simulink model "sldemo_varsize_multimode"  (Simulink 7.6)
settings: Solver=FixedStepDiscrete  StartTime=0.0  StopTime=20  RelTol=1e-3
libraries: simulink x4
settings Model: Creator=The MathWorks Inc.
settings OptimizationCC: InitFltsAndDblsToZero=on
settings SFSimCC: SimParseCustomCode=off

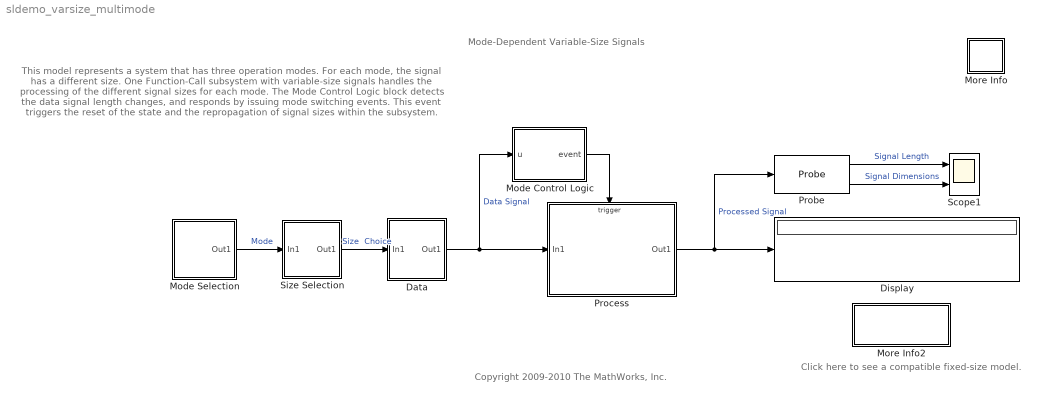
== system sldemo_varsize_multimode ==
  note: Mode-Dependent Variable-Size Signals
  note: Copyright 2009-2010 The MathWorks, Inc.
  note: This model represents a system that has three operation modes. For each mode, the signal has a different size.
      | One Function-Call subsystem with variable-size signals handles the processing of the different signal sizes for each mode. The
      | Mode Control Logic block detects the data signal length changes, and responds by issuing mode switching events. This event
      | triggers the reset of the state and the repropagation of signal sizes within the subsystem.
  note: Click here to see a compatible
      | fixed-size model.
  Data : Subsystem
  Display : Display
  Mode Control Logic : Stateflow chart  TreatAsAtomicUnit=on
  "Mode Selection " : Subsystem
  More Info : Subsystem
      settings: OpenFcn=showdemo(bdroot(gcb))
      mask Display: disp('?')
  More Info2 : Subsystem
      settings: OpenFcn=sldemo_varsize_multimodeFixSizeImpl
      mask Display: disp('Fixed-Size Signal\nImplementation')
  Probe : Probe  ProbeSampleTime=off  ProbeComplexSignal=off  ProbeSignalDimensions=on
  Process : Subsystem  TreatAsAtomicUnit=on
  Scope1 : Scope  NumInputPorts=2
      settings: TimeRange=20  YMin=0~0.5  YMax=10~3.5
  Size Selection : Subsystem
  wires:
  Data/1(Out1) -> Mode Control Logic/1(u), Process/1(In1)  "Data Signal"
  "Mode Selection "/1(Out1) -> Size Selection/1(In1)  "Mode"
  Size Selection/1(Out1) -> Data/1(In1)  "Size  Choice"
  Probe/1 -> Scope1/1  "Signal Length"
  Mode Control Logic/1(event) -> Process/Trigger
  Probe/2 -> Scope1/2  "Signal Dimensions"
  Process/1(Out1) -> Display/1, Probe/1  "Processed Signal"

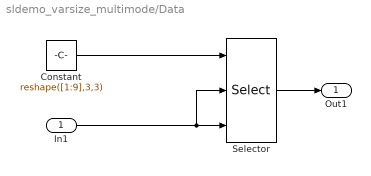
== system sldemo_varsize_multimode/Data ==
  In1 : Inport
  Constant : Constant  Value=reshape([1:9],3,3)
  Selector : Selector  NumberOfDimensions=2  InputPortWidth=3  IndexOptions=Starting and ending indices (port),Starting and ending indices (port)  Indices=[1 3],1  OutputSizes=1,1
  Out1 : Outport
  wires:
  Constant/1 -> Selector/1
  Selector/1 -> Out1/1
  In1/1 -> Selector/3, Selector/2

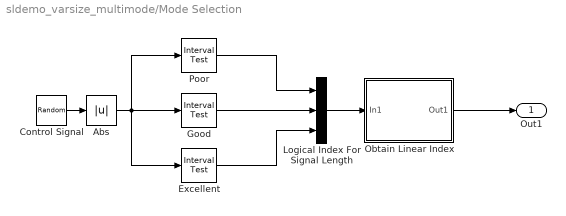
== system sldemo_varsize_multimode/Mode Selection  ==
  Abs : Abs
  Control Signal : RandomNumber  Variance=0.25  SampleTime=1
  Excellent : simulink/Logic and Bit Operations/Interval Test  SystemSampleTime=-1  IntervalClosedRight=off  uplimit=inf  IntervalClosedLeft=on  lowlimit=0.50  LogicOutDataTypeMode=uint8
  Good : simulink/Logic and Bit Operations/Interval Test  SystemSampleTime=-1  IntervalClosedRight=off  uplimit=0.50  IntervalClosedLeft=on  lowlimit=0.25  LogicOutDataTypeMode=uint8
  Logical Index For Signal Length : Concatenate  NumInputs=3  Mode=Vector
  Obtain Linear Index : Subsystem
  Poor : simulink/Logic and Bit Operations/Interval Test  SystemSampleTime=-1  IntervalClosedRight=off  uplimit=0.25  IntervalClosedLeft=on  lowlimit=0.0  LogicOutDataTypeMode=uint8
  Out1 : Outport
  wires:
  Logical Index For Signal Length/1 -> Obtain Linear Index/1(In1)
  Poor/1 -> Logical Index For Signal Length/1
  Excellent/1 -> Logical Index For Signal Length/3
  Good/1 -> Logical Index For Signal Length/2
  Abs/1 -> Excellent/1, Poor/1, Good/1
  Obtain Linear Index/1(Out1) -> Out1/1
  Control Signal/1 -> Abs/1

== system sldemo_varsize_multimode/More Info ==
  note: Bus Block Demonstration
  note: This demonstration shows how signals may be grouped and ungrouped while
      | retaining their names.  In this demonstration, 5 signals are created and labelled
      | appropriately.  These signals are then mux'd together to create a bus of signals.
      | This bus of signals is then fed into the Bus Selector block.  Inside of the Bus
      | Selector block, the Pulse and Chirp signals are chosen to be output from the
      | original signal bus.
      |
      | It is possible to place a nest signal buses and then still retrieve the original signal
      | with its label.

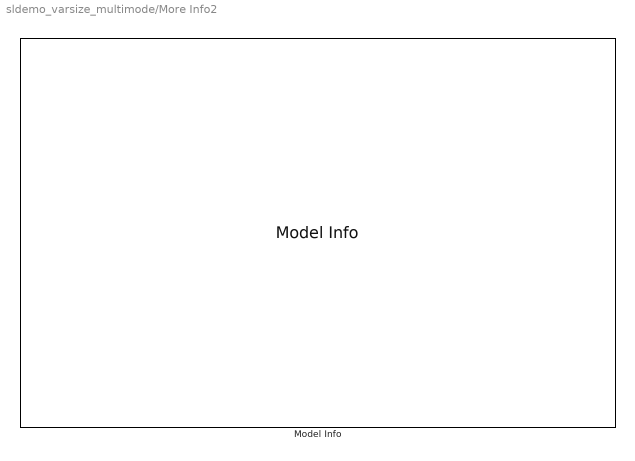
== system sldemo_varsize_multimode/More Info2 ==
  Model Info : simulink/Model-Wide Utilities/Model Info  SystemSampleTime=-1  InitialBlockCM=None  BlockCM=none  Frame=on  DisplayStringWithTags=Model Info  HorizontalTextAlignment=Left  LeftAlignmentValue=0.02  SourceBlockDiagram=sldemo_varsize_multimode  TagMaxNumber=20

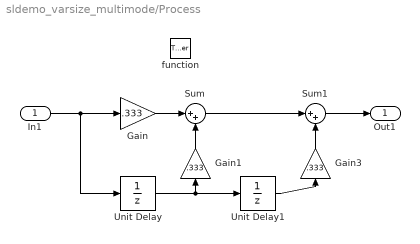
== system sldemo_varsize_multimode/Process ==
  In1 : Inport
  function : TriggerPort  TriggerType=function-call  StatesWhenEnabling=reset  PropagateVarSize=Only when enabling  SampleTimeType=periodic
  Gain : Gain  Gain=.333
  Gain1 : Gain  Gain=.333
  Gain3 : Gain  Gain=.333
  Sum : Sum  Inputs=|++
  Sum1 : Sum  Inputs=|++
  Unit Delay : UnitDelay  SampleTime=-1
  Unit Delay1 : UnitDelay  SampleTime=-1
  Out1 : Outport
  wires:
  Unit Delay/1 -> Gain1/1, Unit Delay1/1
  Gain/1 -> Sum/1
  Gain1/1 -> Sum/2
  In1/1 -> Gain/1, Unit Delay/1
  Unit Delay1/1 -> Gain3/1
  Gain3/1 -> Sum1/2
  Sum/1 -> Sum1/1
  Sum1/1 -> Out1/1

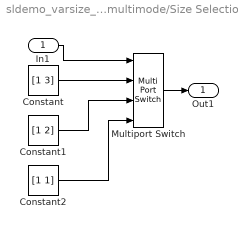
== system sldemo_varsize_multimode/Size Selection ==
  In1 : Inport
  Constant : Constant  Value=[1 3]
  Constant1 : Constant  Value=[1 2]
  Constant2 : Constant  Value=[1 1]
  Multiport Switch : MultiPortSwitch  zeroidx=off
  Out1 : Outport
  wires:
  Constant/1 -> Multiport Switch/2
  Constant1/1 -> Multiport Switch/3
  Constant2/1 -> Multiport Switch/4
  In1/1 -> Multiport Switch/1
  Multiport Switch/1 -> Out1/1

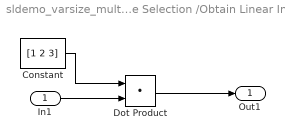
== system sldemo_varsize_multimode/Mode Selection /Obtain Linear Index ==
  In1 : Inport
  Constant : Constant  Value=[1 2 3]
  Dot Product : DotProduct  OutDataTypeStr=Inherit: Inherit via internal rule
  Out1 : Outport
  wires:
  Constant/1 -> Dot Product/1
  Dot Product/1 -> Out1/1
  In1/1 -> Dot Product/2

== stateflow chart Mode Control Logic ==
  settings: updateMethod=DISCRETE  sampleTime=1
  state S
    entry: event;
    during: event;
    bind: event
  (default) -> S
  S -> S : [size_detect()]
  data: y function_output double; u input double
  events: event output FUNCTION_CALL_EVENT
  function y = size_detect:
    | function y = size_detect
    | % Detect signal size changes.
    | % When the input signal size changes the output is set to 1, otherwise it 
    | % is 0.
    | 
    | persistent prevSize;
    | 
    | if isempty(prevSize)
    |    prevSize = 0; 
    | end
    | 
    | if length(u(:)) ~= prevSize
    |     prevSize = length(u(:));
    |     y = 1;
    | else
    |     y = 0;
    | end
